simulink model "saturation_2016"  (R2016b)
settings: Solver=VariableStepAuto  StartTime=0.0  StopTime=10.0  RelTol=1e-3
settings Model: Creator=AKSHAY JP PAWAR  LastModifiedBy=AKSHAY JP PAWAR
settings DataIOCC: ReturnWorkspaceOutputs=on
settings SFSimCC: SimUseLocalCustomCode=on
settings RTWCC: RTWUseLocalCustomCode=on

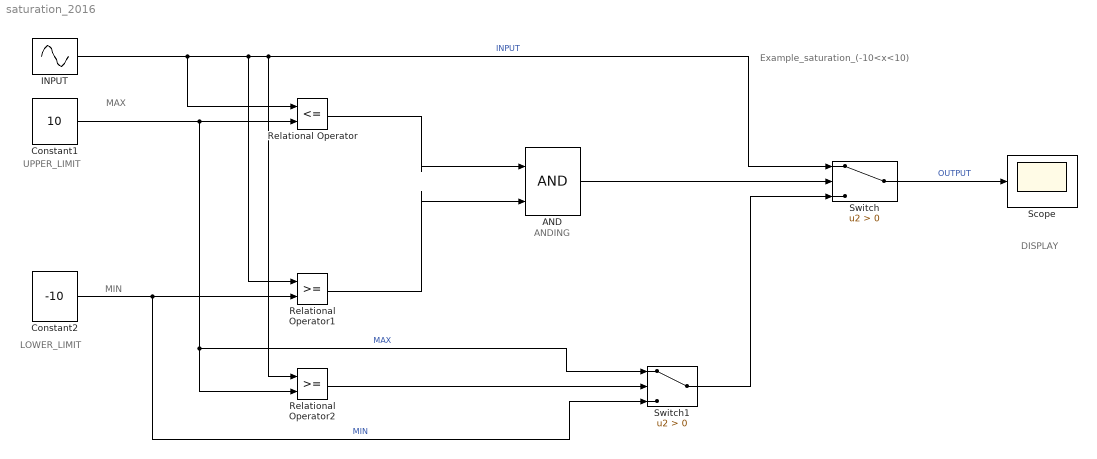
== system saturation_2016 ==
  note: ANDING
  note: MIN
  note: MAX
  note: Example_saturation_(-10<x<10)
  note: DISPLAY
  note: LOWER_LIMIT
  note: UPPER_LIMIT
  AND : Logic  IconShape=distinctive  AllPortsSameDT=off  OutDataTypeStr=boolean
  Constant1 : Constant  Value=10
  Constant2 : Constant  Value=-10
  INPUT : Sin  Amplitude=15  SampleTime=0
  Relational Operator : RelationalOperator  Operator=<=  OutDataTypeStr=boolean  RndMeth=Simplest
  Relational Operator1 : RelationalOperator  OutDataTypeStr=boolean  RndMeth=Simplest
  Relational Operator2 : RelationalOperator  OutDataTypeStr=boolean  RndMeth=Simplest
  Scope : Scope
  Switch : Switch  Criteria=u2 > Threshold
  Switch1 : Switch  Criteria=u2 > Threshold
  wires:
  Constant1/1 -> Switch1/1, Relational Operator2/2, Relational Operator/2  "MAX"
  Relational Operator/1 -> AND/1
  Relational Operator1/1 -> AND/2
  Switch1/1 -> Switch/3
  Switch/1 -> Scope/1  "OUTPUT"
  Constant2/1 -> Relational Operator1/2, Switch1/3  "MIN"
  Relational Operator2/1 -> Switch1/2
  AND/1 -> Switch/2
  INPUT/1 -> Switch/1, Relational Operator2/1, Relational Operator1/1, Relational Operator/1  "INPUT"
